simulink model "RL_nelinearni_model_njihalaCont"  (R2023a)
settings: Solver=FixedStepAuto  StartTime=0.0  StopTime=10  FixedStep=0.01  MaxStep=0.01  RelTol=1e-3
values from neighbouring files (symbols this model uses):
  b1 = 8.3336*10^(-5)    (= 8.3336e-05)    [rl_training.m]
  b2 = 2.5*10^(-4)    (= 0.00025)    [rl_training.m]
  ce = 0.02559    [rl_training.m]
  cm = 0.02559    [rl_training.m]
  g = 9.81    [rl_training.m]
  J0_kapa = 5.5351*10^(-4)    (= 0.00055351)    [rl_training.m]
  J2_kapa = 3.8533*10^(-4)    (= 0.00038533)    [rl_training.m]
  L1 = 10.85*10^(-2)    (= 0.1085)    [rl_training.m]
  l2 = 13.8*10^(-2)    (= 0.138)    [rl_training.m]
  m2 = 18.1*10^(-3)    (= 0.0181)    [rl_training.m]
  n = 3.9    [rl_training.m]
  Ra = 2.19    [rl_training.m]
libraries: simulink x2, rllib x1
settings Model: Creator=Luka  LastModifiedBy=vedran
settings OptimizationCC: ReuseModelBlockBuffer=off
settings HardwareCC: ProdBitPerLong=64  ProdHWDeviceType=Intel->x86-64 (Linux 64)
settings ModelReferenceCC: EnableRefExpFcnMdlSchedulingChecks=on
settings RTWCC: Description=Simulink Desktop Real-Time  SystemTargetFile=sldrt.tlc  TemplateMakefile=sldrt.tmf  RTWCompilerOptimization=on
settings CodeAppCC: MaxIdLength=95
settings SimulinkDesktopRealTimeCC: TargetLibSuffix=_sldrt.a  TargetPreCompLibLocation=C:\Program Files\MATLAB\R2023a\toolbox\sldrt\lib\win64

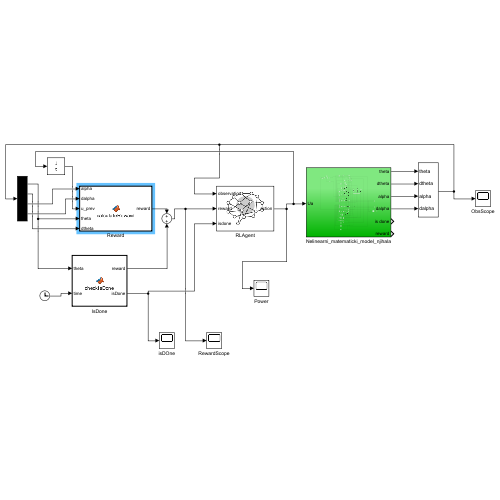
[thumbnail: Simulink's stored preview of the top-level diagram]
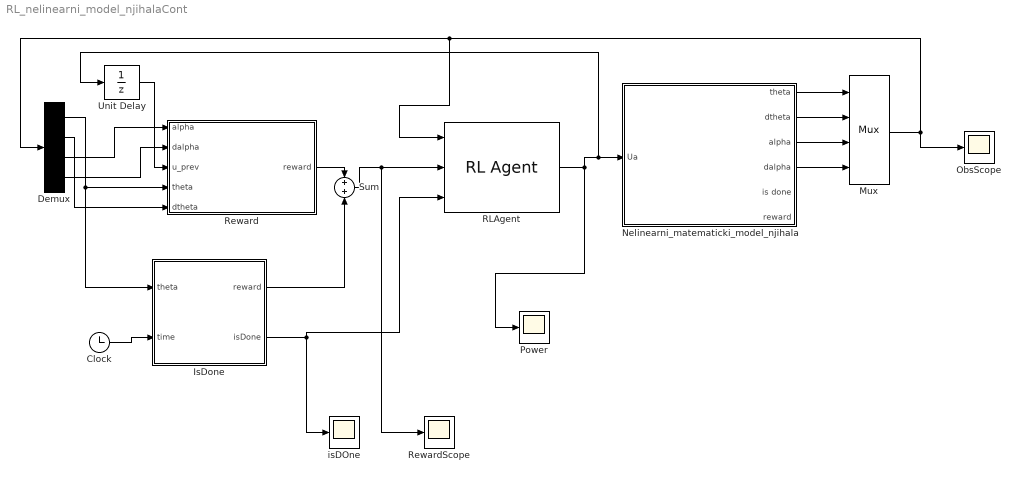
== system RL_nelinearni_model_njihalaCont ==
  Clock : Clock
      settings: Decimation=20
  Demux : Demux
  IsDone : MATLAB Function  TreatAsAtomicUnit=on
  Mux : Mux
      settings: DisplayOption=signals
  Nelinearni_matematicki_model_njihala : Subsystem
  ObsScope : Scope
  Power : Scope
  RLAgent : rllib/RL Agent  Agent=agent  ExternalActionAsInput=off  ProvideLastAction=off  ProvideCumRwd=off  TreatAsDirectFeedthrough=on  UseStrictObservationDataTypes=off
  Reward : MATLAB Function  TreatAsAtomicUnit=on
  RewardScope : Scope
  Sum : Sum
  Unit Delay : UnitDelay  SampleTime=-1  HasFrameUpgradeWarning=on
  isDOne : Scope
  wires:
  Nelinearni_matematicki_model_njihala/1(theta) -> Mux/1
  Nelinearni_matematicki_model_njihala/2(dtheta) -> Mux/2
  Nelinearni_matematicki_model_njihala/3(alpha) -> Mux/3
  Nelinearni_matematicki_model_njihala/4(dalpha) -> Mux/4
  Mux/1 -> Demux/1, RLAgent/1, ObsScope/1
  RLAgent/1 -> Power/1, Unit Delay/1, Nelinearni_matematicki_model_njihala/1(Ua)
  IsDone/1(reward) -> Sum/2
  Reward/1(reward) -> Sum/1
  Sum/1 -> RewardScope/1, RLAgent/2
  IsDone/2(isDone) -> RLAgent/3, isDOne/1
  Clock/1 -> IsDone/2(time)
  Demux/1 -> IsDone/1(theta), Reward/4(theta)
  Demux/3 -> Reward/1(alpha)
  Unit Delay/1 -> Reward/3(u_prev)
  Demux/4 -> Reward/2(dalpha)
  Demux/2 -> Reward/5(dtheta)

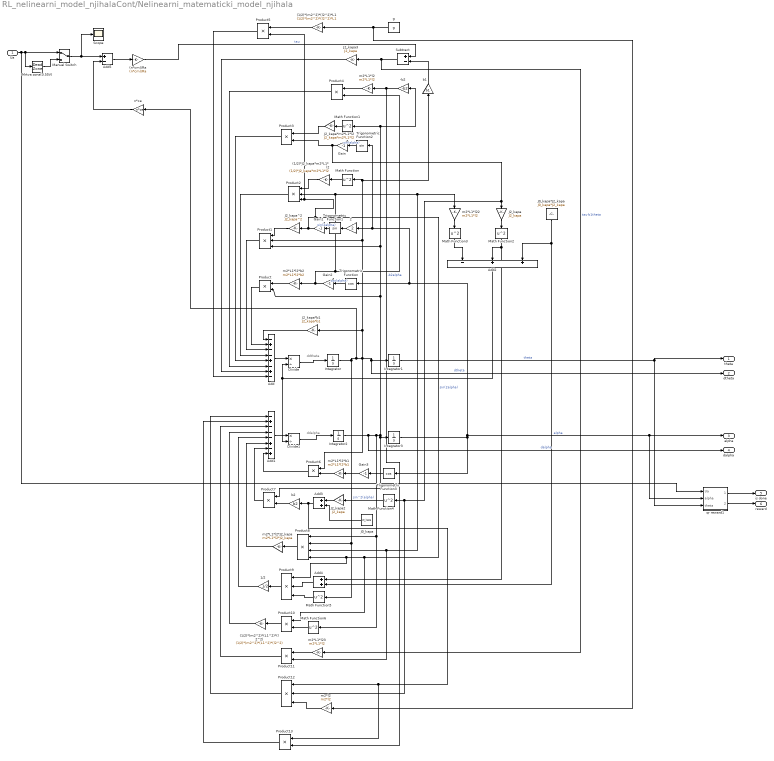
== system RL_nelinearni_model_njihalaCont/Nelinearni_matematicki_model_njihala ==
  note: ddtheta
  note: ddalpha
  Ua : Inport
  (1/2)*(m2^2)*(L1^2)*(l2^2) : Gain  Gain=(1/2)*(m2^2)*(L1^2)*(l2^2)
  (1/2)*(m2^2)*(l2^2)*L1 : Gain  Gain=(1/2)*(m2^2)*(l2^2)*L1
  (1/2)*J2_kapa*m2*L1*l2 : Gain  Gain=(1/2)*J2_kapa*m2*L1*l2
  (n*cm)/Ra : Gain  Gain=(n*cm)/Ra
  -b2 : Gain  Gain=-b2
  1/2 : Gain  Gain=1/2
  2 : Gain  Gain=2
  Add : Sum  Inputs=-+--+-+-
  Add1 : Sum  Inputs=-+---+-+
  Add2 : Sum  Inputs=-++
  Add3 : Sum
  Add4 : Sum
  Add5 : Sum  Inputs=+-
  Divide : Product  Inputs=*/
  Divide1 : Product  Inputs=*/
  Gain{,1..3} (4 alike) : Gain  Gain=-1
  Integrator : Integrator
  Integrator1 : Integrator
  Integrator2 : Integrator  InitialCondition=(rand()*5)-2.5
  Integrator3 : Integrator  InitialCondition=(rand()*2*pi)-pi
  J0_kapa : Constant  Value=J0_kapa
  J0_kapa*J2_kapa : Constant  Value=J0_kapa*J2_kapa
  J2_kapa : Gain  Gain=J2_kapa
  J2_kapa*b1 : Gain  Gain=J2_kapa*b1
  J2_kapa*m2*L1*l2 : Gain  Gain=J2_kapa*m2*L1*l2
  J2_kapa2 : Gain  Gain=J2_kapa
  J2_kapa3 : Gain  Gain=J2_kapa
  J2_kapa^2 : Gain  Gain=J2_kapa^2
  Manual Switch : ManualSwitch
  Math Function{,1..6} (7 alike) : Math  Operator=square
  Mrtva zona(0.55V) : DeadZone  LowerValue=-0.55  UpperValue=0.55
  Product{,3..7,10..11,13} (9 alike) : Product
  Product{1..2,9,12} (4 alike) : Product  Inputs=3
  Product8 : Product  Inputs=4
  Scope : Scope
  Subtract : Sum  Inputs=+-
  Trigonometric Function : Trigonometry  Operator=cos
  Trigonometric Function1 : Trigonometry
  Trigonometric Function2 : Trigonometry
  Trigonometric Function3 : Trigonometry  Operator=cos
  b1 : Gain  Gain=b1
  b2 : Gain  Gain=b2
  g : Constant  Value=g
  m2*L1*l2 : Gain  Gain=m2*L1*l2
  m2*L1*l2*J2_kapa : Gain  Gain=m2*L1*l2*J2_kapa
  m2*L1*l2*b1 : Gain  Gain=m2*L1*l2*b1
  m2*L1*l2*b2 : Gain  Gain=m2*L1*l2*b2
  m2*L1*l22 : Gain  Gain=m2*L1*l2
  m2*L1*l23 : Gain  Gain=m2*L1*l2
  m2*l2 : Gain  Gain=m2*l2
  n*ce : Gain  Gain=n*ce
  qr reward1 : Subsystem
  theta : Outport
  dtheta : Outport  Port=2
  alpha : Outport  Port=3
  dalpha : Outport  Port=4
  is done : Outport  Port=5  VectorParamsAs1DForOutWhenUnconnected=off
  reward : Outport  Port=6  VectorParamsAs1DForOutWhenUnconnected=off
  wires:
  Add4/1 -> Product9/2
  Add3/1 -> Product13/1, Product12/1, b2/1
  Trigonometric Function2/1 -> Gain/1  "sin(alpha)"
  Product3/1 -> Add/5
  m2*L1*l2*J2_kapa/1 -> Add1/6
  Add1/1 -> Divide1/1
  m2*L1*l2/1 -> Product4/1
  Add2/1 -> Divide1/2, Divide/2
  Trigonometric Function/1 -> Gain2/1  "cos(alpha)"
  m2*L1*l2*b2/1 -> Product/1
  Integrator/1 -> n*ce/1, Product6/1, b1/1, Math Function/1, Product1/2, J2_kapa*b1/1, dtheta/1, Integrator1/1, Math Function5/1, Product8/2  "dtheta"
  Math Function3/1 -> Add2/1
  Product10/1 -> (1/2)*(m2^2)*(L1^2)*(l2^2)/1
  Divide1/1 -> Integrator2/1
  m2*l2/1 -> Product12/3
  Integrator2/1 -> dalpha/1, Math Function6/1, Product8/1, Integrator3/1, Product7/1, -b2/1, Math Function1/1, Product1/3, Product/2  "dalpha"
  J2_kapa*b1/1 -> Add/1
  m2*L1*l2*b1/1 -> Product6/2
  2/1 -> Trigonometric Function1/1
  Gain1/1 -> J2_kapa^2/1, Product10/1, Product9/1, Product8/4, Product5/2, Product2/3  "sin(2alpha)"
  J2_kapa3/1 -> Add/7
  J2_kapa^2/1 -> Product1/1
  Product1/1 -> Add/3
  (1/2)*(m2^2)*(L1^2)*(l2^2)/1 -> Add1/4
  Product5/1 -> Add/8
  Math Function1/1 -> J2_kapa*m2*L1*l2/1
  (1/2)*(m2^2)*(l2^2)*L1/1 -> Product5/1
  m2*L1*l23/1 -> Product11/1
  Product/1 -> Add/2
  J0_kapa/1 -> Add3/2
  J0_kapa*J2_kapa/1 -> Add4/2, Add2/3
  Product4/1 -> Add/6
  Add/1 -> Divide/1
  J2_kapa2/1 -> Add3/1
  Product7/1 -> Add1/7
  g/1 -> (1/2)*(m2^2)*(l2^2)*L1/1, m2*l2/1
  Math Function4/1 -> J2_kapa2/1  "sin^2(alpha)"
  J2_kapa/1 -> Math Function2/1
  Divide/1 -> Integrator/1
  m2*L1*l22/1 -> Math Function3/1
  Math Function/1 -> (1/2)*J2_kapa*m2*L1*l2/1
  1/2/1 -> Add1/5
  Product2/1 -> Add/4
  Math Function2/1 -> Add4/1, Add2/2
  (1/2)*J2_kapa*m2*L1*l2/1 -> Product2/1
  Product12/1 -> Add1/1
  Product8/1 -> m2*L1*l2*J2_kapa/1
  Integrator1/1 -> theta/1, qr reward1/3(theta)  "theta"
  Product6/1 -> Add1/8
  Product9/1 -> 1/2/1
  Math Function5/1 -> Product9/3
  Product11/1 -> Add1/3
  (n*cm)/Ra/1 -> Subtract/1  "tau"
  Math Function6/1 -> Product10/2
  J2_kapa*m2*L1*l2/1 -> Product3/1
  -b2/1 -> Product13/2, m2*L1*l2/1  "-b2alpha"
  Trigonometric Function3/1 -> Gain3/1
  b2/1 -> Product7/2
  n*ce/1 -> Add5/2
  Add5/1 -> (n*cm)/Ra/1
  b1/1 -> Subtract/2
  Subtract/1 -> J2_kapa3/1, m2*L1*l23/1  "tau-b1theta"
  Product13/1 -> Add1/2
  Gain/1 -> Product12/2, Math Function4/1, J2_kapa/1, Product3/2
  Trigonometric Function1/1 -> Gain1/1  "sin(2alpha)"
  Gain2/1 -> m2*L1*l2*b2/1, Product4/2, Product11/2, Product8/3, m2*L1*l22/1, Product2/2
  Gain3/1 -> m2*L1*l2*b1/1
  Manual Switch/1 -> Scope/1, Add5/1
  Mrtva zona(0.55V)/1 -> Manual Switch/2
  Integrator3/1 -> Trigonometric Function2/1, 2/1, Trigonometric Function/1, qr reward1/2(alpha), alpha/1, Trigonometric Function3/1  "alpha"
  qr reward1/1(is done) -> is done/1
  Ua/1 -> qr reward1/1(Ua), Mrtva zona(0.55V)/1, Manual Switch/1
  qr reward1/2(reward) -> reward/1

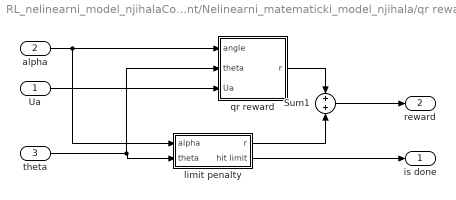
== system RL_nelinearni_model_njihalaCont/Nelinearni_matematicki_model_njihala/qr reward1 ==
  Ua : Inport
  alpha : Inport  Port=2
  theta : Inport  Port=3
  Sum1 : Sum
  limit penalty : Subsystem
  qr reward : Subsystem
  is done : Outport  VectorParamsAs1DForOutWhenUnconnected=off
  reward : Outport  Port=2  VectorParamsAs1DForOutWhenUnconnected=off
  wires:
  Sum1/1 -> reward/1
  qr reward/1(r) -> Sum1/1
  limit penalty/2(hit limit) -> is done/1
  theta/1 -> limit penalty/2(theta), qr reward/2(theta)
  alpha/1 -> limit penalty/1(alpha), qr reward/1(angle)
  Ua/1 -> qr reward/3(Ua)
  limit penalty/1(r) -> Sum1/2

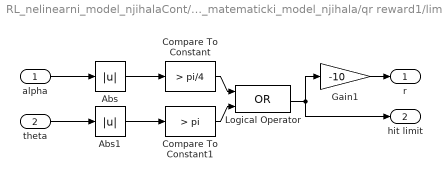
== system RL_nelinearni_model_njihalaCont/Nelinearni_matematicki_model_njihala/qr reward1/limit penalty ==
  alpha : Inport
  theta : Inport  Port=2
  Abs : Abs  SaturateOnIntegerOverflow=off
  Abs1 : Abs  SaturateOnIntegerOverflow=off
  Compare To Constant : simulink/Logic and Bit Operations/Compare To Constant  relop=>  const=pi/4  OutDataTypeStr=boolean
  Compare To Constant1 : simulink/Logic and Bit Operations/Compare To Constant  relop=>  const=pi  OutDataTypeStr=boolean
  Gain1 : Gain  Gain=-10
  Logical Operator : Logic  Operator=OR  AllPortsSameDT=off  OutDataTypeStr=boolean
  r : Outport  VectorParamsAs1DForOutWhenUnconnected=off
  hit limit : Outport  Port=2  VectorParamsAs1DForOutWhenUnconnected=off
  wires:
  Gain1/1 -> r/1
  alpha/1 -> Abs/1
  Abs/1 -> Compare To Constant/1
  Logical Operator/1 -> hit limit/1, Gain1/1
  Abs1/1 -> Compare To Constant1/1
  theta/1 -> Abs1/1
  Compare To Constant1/1 -> Logical Operator/2
  Compare To Constant/1 -> Logical Operator/1

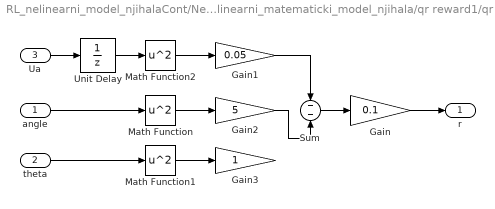
== system RL_nelinearni_model_njihalaCont/Nelinearni_matematicki_model_njihala/qr reward1/qr reward ==
  angle : Inport
  theta : Inport  Port=2
  Ua : Inport  Port=3
  Gain : Gain  Gain=0.1
  Gain1 : Gain  Gain=0.05
  Gain2 : Gain  Gain=5
  Gain3 : Gain
  Math Function : Math  Operator=square  SignedPower=on
  Math Function1 : Math  Operator=square  SignedPower=on
  Math Function2 : Math  Operator=square  SignedPower=on
  Sum : Sum  Inputs=--
  Unit Delay : UnitDelay  SampleTime=-1  HasFrameUpgradeWarning=on
  r : Outport  VectorParamsAs1DForOutWhenUnconnected=off
  wires:
  angle/1 -> Math Function/1
  Gain2/1 -> Sum/2
  Math Function2/1 -> Gain1/1
  Math Function1/1 -> Gain3/1
  theta/1 -> Math Function1/1
  Math Function/1 -> Gain2/1
  Gain1/1 -> Sum/1
  Sum/1 -> Gain/1
  Ua/1 -> Unit Delay/1
  Gain/1 -> r/1
  Unit Delay/1 -> Math Function2/1

== matlab function RL_nelinearni_model_njihalaCont/IsDone ==
  data: reward output; theta input; isDone output; time input
function [reward, isDone]= checkIsDone(theta , time)
    thetalimit = pi/2;
    timeLimit = 10;
    if abs(theta) > thetalimit
        reward = -10;
        isDone = true;
    elseif time >= timeLimit
        reward = 0;
        isDone = true;
    else
        reward = 0;
        isDone = false;
    end
end

== matlab function RL_nelinearni_model_njihalaCont/Reward ==
  data: alpha input; dalpha input; u_prev input; reward output; theta input; dtheta input
function reward = calculateReward(alpha, dalpha, u_prev, theta, dtheta)
    alpha_wrapped = wrapToPi(alpha);
    active_reward =   - (alpha_wrapped^2 + 0.01*dalpha^2 + 0.01*theta^2 + 0.001*u_prev^2);
    if alpha_wrapped < pi/8
        balancing_reward = 1;
        reward = active_reward + balancing_reward;
    else
        reward = active_reward;
    end
end
